simulink model "system_sim"  (R2023b)
settings: Solver=VariableStepAuto  StartTime=0.0  StopTime=10  RelTol=1e-3
values from neighbouring files (symbols this model uses):
  ct_A = rp_sys.A    [system_load.m]
  ct_B = rp_sys.B    [system_load.m]
  ct_C = [1 0 0 0 ... (first row only)    [system_load.m]
  ct_D = [0; 0]    [system_load.m]
  F = dt_A - L * dt_C - dt_B * K    [system_load.m]
  G = L    [system_load.m]
  H = -K    [system_load.m]
  J = [0 0]    [system_load.m]
  ts = 0.02    [system_load.m]
  xp_init = [0.1; 0.04; 0; 0]    [system_load.m]
settings Model: Creator=mike5  LastModifiedBy=mike5

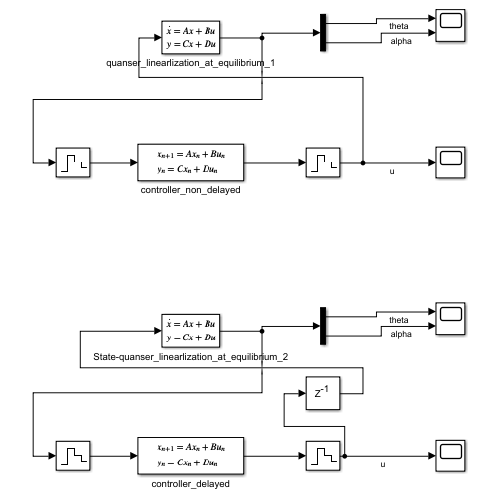
[thumbnail: Simulink's stored preview of the top-level diagram]
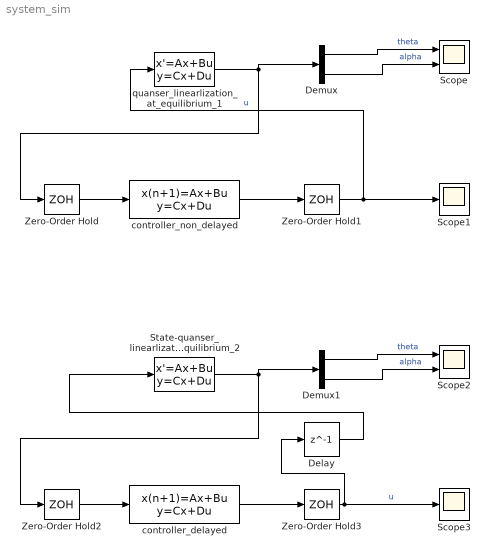
== system system_sim ==
  Delay : Delay  DelayLength=1  InitialCondition=0
  Demux : Demux  Outputs=2
  Demux1 : Demux  Outputs=2
  Scope : Scope  NumInputPorts=2
  Scope1 : Scope
  Scope2 : Scope  NumInputPorts=2
  Scope3 : Scope
  State-quanser_linearlization_at_equilibrium_2 : StateSpace  A=ct_A  B=ct_B  C=ct_C  D=ct_D  InitialCondition=xp_init
  Zero-Order Hold : ZeroOrderHold  SampleTime=ts
  Zero-Order Hold1 : ZeroOrderHold  SampleTime=-1
  Zero-Order Hold2 : ZeroOrderHold  SampleTime=ts
  Zero-Order Hold3 : ZeroOrderHold  SampleTime=-1
  controller_delayed : DiscreteStateSpace  A=F  B=G  C=H  D=J  SampleTime=-1
  controller_non_delayed : DiscreteStateSpace  A=F  B=G  C=H  D=J  SampleTime=-1
  quanser_linearlization_at_equilibrium_1 : StateSpace  A=ct_A  B=ct_B  C=ct_C  D=ct_D  InitialCondition=xp_init
  wires:
  Zero-Order Hold/1 -> controller_non_delayed/1
  controller_non_delayed/1 -> Zero-Order Hold1/1
  quanser_linearlization_at_equilibrium_1/1 -> Demux/1, Zero-Order Hold/1
  Zero-Order Hold1/1 -> quanser_linearlization_at_equilibrium_1/1, Scope1/1  "u"
  Demux/1 -> Scope/1  "theta"
  Demux/2 -> Scope/2  "alpha"
  State-quanser_linearlization_at_equilibrium_2/1 -> Demux1/1, Zero-Order Hold2/1
  Zero-Order Hold3/1 -> Delay/1, Scope3/1  "u"
  Demux1/2 -> Scope2/2  "alpha"
  Demux1/1 -> Scope2/1  "theta"
  Zero-Order Hold2/1 -> controller_delayed/1
  controller_delayed/1 -> Zero-Order Hold3/1
  Delay/1 -> State-quanser_linearlization_at_equilibrium_2/1
